simulink model "Ex3_Function_Compute"  (R2017a)
settings: Solver=VariableStepAuto  StartTime=-3*pi  StopTime=3*pi  RelTol=1e-3
settings Model: Creator=sulaymon.eshkabilov  LastModifiedBy=sulaymon.eshkabilov

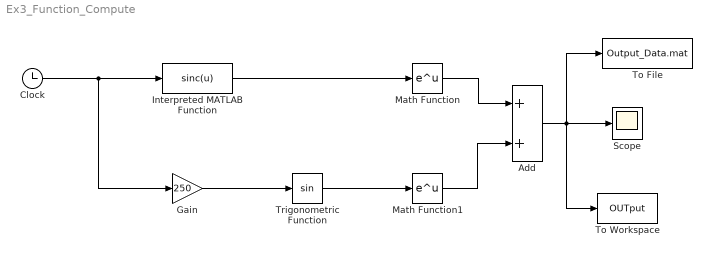
== system Ex3_Function_Compute ==
  Add : Sum
  Clock : Clock
  Gain : Gain  Gain=250
  Interpreted MATLAB Function : MATLABFcn  MATLABFcn=sinc(u)
  Math Function : Math  SaturateOnIntegerOverflow=on
  Math Function1 : Math  SaturateOnIntegerOverflow=on
  Scope : Scope
  To File : ToFile  Filename=Output_Data.mat  SaveFormat=Timeseries
  To Workspace : ToWorkspace  VariableName=OUTput  SaveFormat=Timeseries  SampleTime=-1
  Trigonometric Function : Trigonometry
  wires:
  Trigonometric Function/1 -> Math Function1/1
  Gain/1 -> Trigonometric Function/1
  Clock/1 -> Interpreted MATLAB Function/1, Gain/1
  Interpreted MATLAB Function/1 -> Math Function/1
  Math Function/1 -> Add/1
  Math Function1/1 -> Add/2
  Add/1 -> To Workspace/1, To File/1, Scope/1
